simulink subsystem "Adaptative_Gain_Controller"  (R2020b)
settings: Solver=VariableStepAuto  StartTime=0.0  StopTime=10.0  RelTol=1e-3
model mask{lambda_0=1, lambda_inf=0, lambda_prime_0=1}
settings Model: Creator=marco  LastModifiedBy=marco

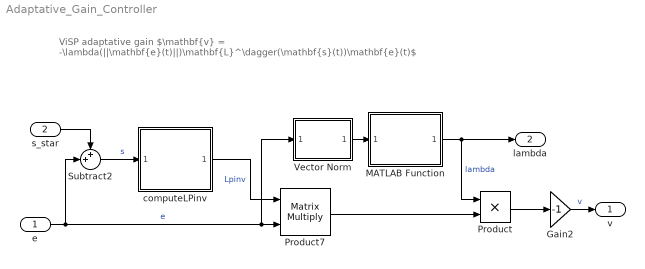
== system Adaptative_Gain_Controller ==
  note: ViSP adaptative gain
      | $\mathbf{v} = -\lambda(||\mathbf{e}(t)||)\mathbf{L}^\dagger(\mathbf{s}(t))\mathbf{e}(t)$
  e : Inport
  s_star : Inport  Port=2
  Gain2 : Gain  Gain=-1
  MATLAB Function : MATLAB Function  TreatAsAtomicUnit=on
  Product : Product
  Product7 : Product  Multiplication=Matrix(*)
  Subtract2 : Sum  Inputs=++|
  Vector Norm : Subsystem  ReferencedSubsystem=Norm
  computeLPinv : Subsystem  ReferencedSubsystem=computeLPinv
  v : Outport
  lambda : Outport  Port=2
  wires:
  Vector Norm/1 -> MATLAB Function/1(norm_e)
  Product/1 -> Gain2/1
  Gain2/1 -> v/1  "v"
  MATLAB Function/1(lambda) -> lambda/1, Product/1  "lambda"
  computeLPinv/1 -> Product7/1  "Lpinv"
  Subtract2/1 -> computeLPinv/1  "s"
  Product7/1 -> Product/2
  e/1 -> Subtract2/2, Vector Norm/1, Product7/2  "e"
  s_star/1 -> Subtract2/1

== matlab function Adaptative_Gain_Controller/MATLAB Function ==
  data: norm_e input; lambda output; lambda_0 parameter; lambda_inf parameter; lambda_prime_0 parameter
function lambda = fcn(norm_e,lambda_0, lambda_inf, lambda_prime_0)

lambda = (lambda_0-lambda_inf)*exp(-lambda_prime_0*norm_e/(lambda_0-lambda_inf)) + lambda_inf;
